simulink subsystem "MotorsDCEquivalentFaulhaber_Variant1"  (R2026a)
settings: Solver=VariableStepAuto
undefined symbols (not defined in the file): Motor1, Motor2, Motor3, Phase1_Pos, Phase2_Pos, Phase3_Pos, Phase_Neg, Reference
libraries: fl_lib x1
settings Model: DataDictionary=neck_mk3.sldd  EnableAccessToBaseWorkspace=off  Creator=upattacini  LastModifiedBy=upattacini

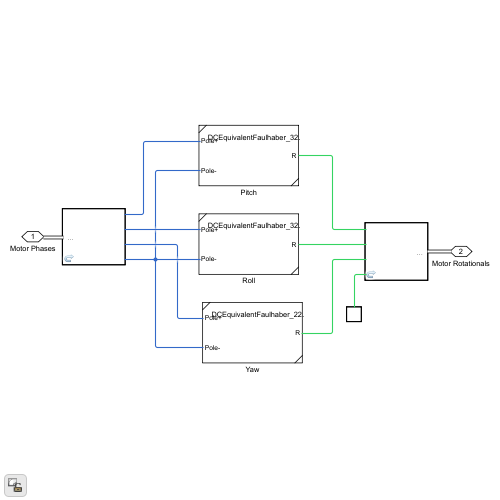
[thumbnail: Simulink's stored preview of the top-level diagram]
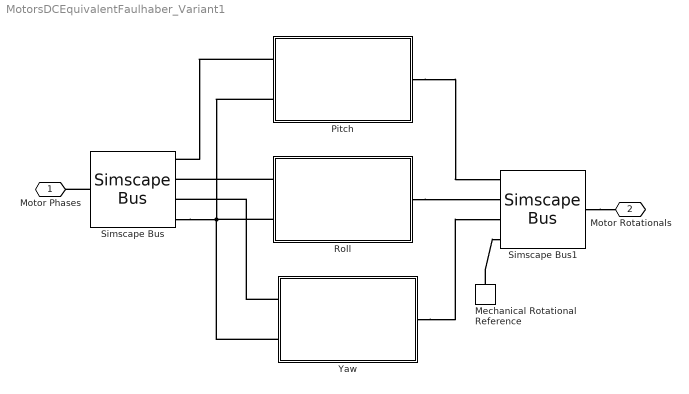
== system MotorsDCEquivalentFaulhaber_Variant1 ==
  Mechanical Rotational Reference : fl_lib/Mechanical/Rotational Elements/Mechanical Rotational Reference
  Pitch : Subsystem  ReferencedSubsystem=DCEquivalentFaulhaber_3216_024_BXTH
      settings: PermitHierarchicalResolution=None
  Roll : Subsystem  ReferencedSubsystem=DCEquivalentFaulhaber_3216_024_BXTH
      settings: PermitHierarchicalResolution=None
  Simscape Bus : SimscapeBus  HierarchyStrings=Phase1_Pos;Phase2_Pos;Phase3_Pos;Phase_Neg  ConnectionType=Bus: Physical_MotorPhases
  Simscape Bus1 : SimscapeBus  HierarchyStrings=Motor1;Motor2;Motor3;Reference  ConnectionType=Bus: Physical_MotorRotationals
  Yaw : Subsystem  ReferencedSubsystem=DCEquivalentFaulhaber_2214_024_BXTH
      settings: PermitHierarchicalResolution=None
  Motor Phases : PMIOPort  Side=Left
  Motor Rotationals : PMIOPort  Port=2  Side=Right
  connections:
  Simscape Bus/LConn4 -- Yaw/LConn2 -- Roll/LConn2 -- Pitch/LConn2
  Simscape Bus/RConn1 -- Motor Phases/RConn1
  Simscape Bus1/RConn1 -- Motor Rotationals/RConn1
  Pitch/RConn1 -- Simscape Bus1/LConn1
  Yaw/RConn1 -- Simscape Bus1/LConn3
  Roll/RConn1 -- Simscape Bus1/LConn2
  Pitch/LConn1 -- Simscape Bus/LConn1
  Roll/LConn1 -- Simscape Bus/LConn2
  Yaw/LConn1 -- Simscape Bus/LConn3
  Mechanical Rotational Reference/LConn1 -- Simscape Bus1/LConn4
